simulink model "04_ee_d"  (R2023a)
settings: Solver=VariableStepDiscrete  StartTime=0.0  StopTime=2  RelTol=1e-3  EnableMultiTasking=on
PreLoadFcn:
  | Pnom=100e6;
  | Vnom=35e3;
  | Fnom=50;        %Hz
  | 
  | %DC link
  | Vdc_nom=70e3;       %Volts
  | C_DClink=200e-6; %Farads
  | 
  | %Choke data
  | R_RL=0.10/100;  %pu
  | L_RL=0.10;      %pu
InitFcn:
  | Ts_Power=5e-6;
  | Ts_Control=50e-6;
  | Ts=5e-6;
  | PWM_freq=2600;
undefined symbols (not defined in the file): D11, Delta, DiscIntNeverNeededParam
libraries: spsParallelRLCBranchLib x2, spsThreePhaseVIMeasurementLib x2, spsabctodq0Lib x2, spsSecondOrderFilterLib x2, simulink_extras x2, spsThreePhaseMutualInductanceZ1Z0Lib x1, spsVoltageMeasurementLib x1, spsThreePhaseProgrammableVoltageSourceLib x1, spsThreePhaseTransformerTwoWindingsLib x1, spsDCVoltageSourceLib x1, spsPLL3phLib x1, spsPowerdq0InstantaneousLib x1
settings Model: SimulationMode=accelerator  Creator=Eric  LastModifiedBy=eagle
settings SolverCC: AlgebraicLoopSolver=TrustRegion
settings DataIOCC: SaveFormat=StructureWithTime  SignalLoggingSaveFormat=ModelDataLogs  SaveOutput=off  SignalLogging=off  SaveTime=off  ReturnWorkspaceOutputs=off
settings OptimizationCC: ExpressionDepthLimit=2147483647  InitFltsAndDblsToZero=on  LifeSpan=inf
settings DebuggingCC: SaveWithParameterizedLinksMsg=none  UnderspecifiedInitializationDetection=Classic  MergeDetectMultiDrivingBlocksExec=none  SignalResolutionControl=TryResolveAllWithWarning  SolverPrmCheckMsg=warning  MultiTaskDSMMsg=warning  MultiTaskCondExecSysMsg=none  FcnCallInpInsideContextMsg=warning  AllowSymbolicDim=off  StateNameClashWarn=warning  SFUnexpectedBacktrackingDiag=warning  SFNoUnconditionalDefaultTransitionDiag=warning  SFExecutionAtInitializationDiag=none  ArithmeticOperatorsInVariantConditions=warning
settings HardwareCC: ProdBitPerPointer=32  ProdBitPerSizeT=32  ProdBitPerPtrDiffT=32  ProdLargestAtomicFloat=None  ProdIntDivRoundTo=Undefined  ProdEndianess=Unspecified  ProdWordSize=32  ProdHWDeviceType=32-bit Generic
settings ModelReferenceCC: EnableRefExpFcnMdlSchedulingChecks=on  PropagateSignalLabelsOutOfModel=off
settings SFSimCC: SimUseLocalCustomCode=off  CustomCodeUndefinedFunction=UseInterfaceOnly
settings RTWCC: RTWUseLocalCustomCode=off
settings CodeAppCC: StateflowObjectComments=on
settings GRTTargetCC: TargetFcnLib=ansi_tfl_tmw.mat  TargetLangStandard=C89/C90 (ANSI)  CombineOutputUpdateFcns=off  GRTInterface=on
settings ConfigComp: CovMetricSettings=dw  CovSaveCumulativeToWorkspaceVar=on  CovSaveSingleToWorkspaceVar=on  CovExternalEMLEnable=off  CovSFcnEnable=off
settings SimscapeCC: SimscapeNormalizeSystem=off

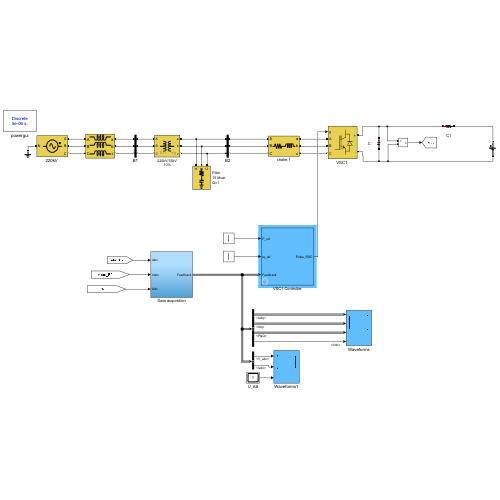
[thumbnail: Simulink's stored preview of the top-level diagram]
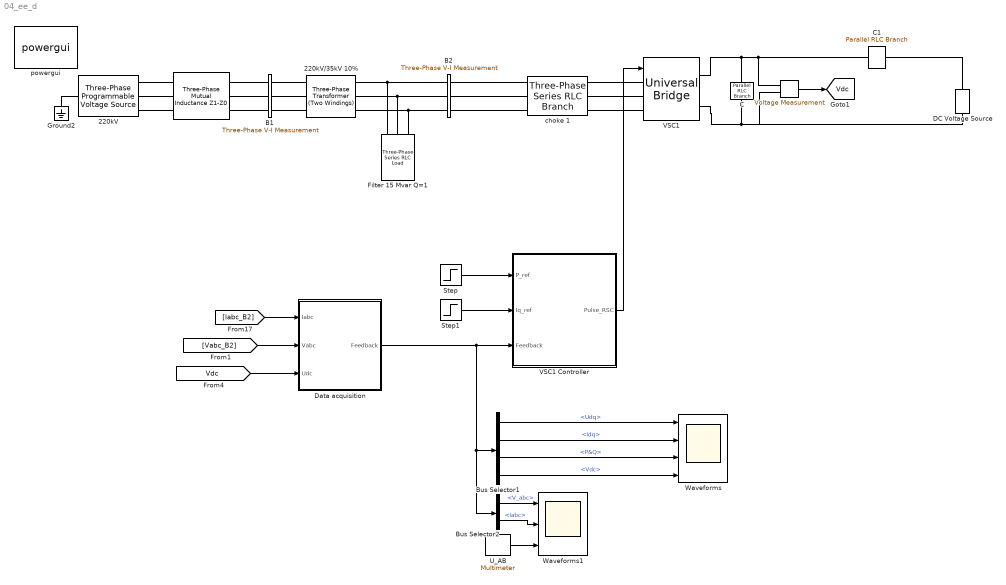
== system 04_ee_d ==
  "  " : spsThreePhaseMutualInductanceZ1Z0Lib/Three-Phase Mutual Inductance Z1-Z0  LConnTagsString=a|b|c  RConnTagsString=A|B|C  PositiveSequence="[ 220e3^2/(10*Pnom)/10  220e3^2/(10*Pnom)/(2*pi*50)]"  ZeroSequence="[220e3^2/(10*Pnom)/10*3  220e3^2/(10*Pnom)/(2*pi*50)*3]"
      settings: AttributesFormatString=\n
      settings: LibrarySourceBlock=|
      | sps_lib/Power Grid Elements/Three-Phase
      | Mutual Inductance
      | Z1-Z0
  "     " : spsVoltageMeasurementLib/Voltage Measurement  PhasorSimulation=off  OutputType=Complex  PSBequivalent=0
  " C" : spsParallelRLCBranchLib/Parallel RLC Branch  LConnTagsString=a  RConnTagsString=__new0  BranchType=C  Resistance=1000000  Inductance=1e-3  SetiL0=off  InitialCurrent=0  Capacitance=C_DClink  Setx0=on  InitialVoltage=Vdc_nom  Measurements=None
  " C1" : spsParallelRLCBranchLib/Parallel RLC Branch  LConnTagsString=a  RConnTagsString=__new0  BranchType=R  Resistance=5  Inductance=1e-3  SetiL0=off  InitialCurrent=0  Capacitance=C_DClink  Setx0=on  InitialVoltage=Vdc_nom  Measurements=None
  "220kV " : spsThreePhaseProgrammableVoltageSourceLib/Three-Phase Programmable Voltage Source  PositiveSequence=[220e3 0 50]  VariationEntity=None  VariationType=Table of time-amplitude pairs  VariationTypeAlt=Step  VariationStep=-0.2  VariationRate=10  VariationMagnitude=0.3  VariationFrequency=2  VariationTiming=[0.05 0.05+5/60]  VariationPhaseA=off  Amplitudes=[1 0.8 1.0]  TimeValues=[0 0.03 0.13]  HarmonicGeneration=off  HarmonicA=[1 0.05 0 2]  HarmonicB=[0 0 0 0]  Timing="[2  20]"  BusType=swing  Pref=0  Qref=0  Qmin=-inf  Qmax=inf
  220kV/35kV 10% : spsThreePhaseTransformerTwoWindingsLib/Three-Phase Transformer (Two Windings)  Winding1Connection=Delta (D11)  Winding2Connection=Yg  CoreType=Three single-phase transformers  SetSaturation=off  Hysteresis=off  DataFile='basic_model'  SetInitialFlux=off  Measurements=None  UNITS=pu  NominalPower=[Pnom*1.5 50 ]  Winding1="[ 220e3  0.05/30   0.05]"  Winding2="[ Vnom 0.05/30  0.05]"  Rm=500  Lm=500  L0=0.5  Saturation="[ 0,0  ;  0.005,1.2  ;  1.0,1.4 ]"  InitialFluxes=[ 0.8 , -0.8 , 0.7 ]  BreakLoop=off  DiscreteSolver=Trapezoidal iterative  DataType=off  TransfoNumber=0
  B1 : spsThreePhaseVIMeasurementLib/Three-Phase V-I Measurement  VoltageMeasurement=phase-to-ground  SetLabelV=on  LabelV=Vabc_B1  Vpu=on  VpuLL=off  CurrentMeasurement=yes  SetLabelI=on  LabelI=Iabc_B1  Ipu=on  Pbase=Pnom  Vbase=220e3  OutputType=Complex  PhasorSimulation=off  PSBequivalent=0
  B2 : spsThreePhaseVIMeasurementLib/Three-Phase V-I Measurement  VoltageMeasurement=phase-to-phase  SetLabelV=on  LabelV=Vabc_B2  Vpu=on  VpuLL=off  CurrentMeasurement=yes  SetLabelI=on  LabelI=Iabc_B2  Ipu=on  Pbase=Pnom  Vbase=Vnom  OutputType=Complex  PhasorSimulation=off  PSBequivalent=0
  Bus Selector1 : BusSelector  OutputSignals=Udq,Idq,P&Q,Vdc
  Bus Selector2 : BusSelector  OutputSignals=V_abc,Iabc
  DC Voltage Source : spsDCVoltageSourceLib/DC Voltage Source  Amplitude=Vdc_nom  Measurements=Voltage
  Data acquisition : Subsystem
  Filter 15 Mvar Q=1 : spsThreePhaseSeriesRLCLoadLib/Three-Phase Series RLC Load  LConnTagsString=A|B|C  Configuration=Y (grounded)  NominalVoltage=Vnom  Vabc=[1e3 1e3 1e3]  Vabcp=[1e3 1e3 1e3]  NominalFrequency=Fnom  UnbalancedPower=off  ActivePower=Pnom*0.15/50  InductivePower=0  CapacitivePower=Pnom*0.15  Pabc=[10e3 9e3 11e3]  QLabc=[100 90 110]  QCabc=[100 90 110]  Pabcp=[10e3 9e3 11e3]  QLabcp=[100 90 110]  QCabcp=[100 90 110]  Measurements=None  LoadType=constant Z
  Ground2 : spsGroundLib/Ground  LConnTagsString=a
  Step : Step  Before=0.5  SampleTime=0
  Step1 : Step  Time=1.5  After=0.2  SampleTime=0
  U_AB : spsMultimeterLib/Multimeter  L=5  sel=1  yselected={}  Gain=1  OutputType=Complex  PlotAtSimulationStop=off  PhasorSimulation=off
  "VSC1 " : spsUniversalBridgeLib/Universal Bridge  Arms=3  SnubberResistance=5000  SnubberCapacitance=1e-6  Device=IGBT / Diodes  Ron=1e-3  Lon=0  ForwardVoltages="[  0  0  ]"  ForwardVoltage=0  GTOparameters=[ 10e-6 , 20e-6 ]  IGBTparameters=[ 0 , 0 ]  Measurements=UAB UBC UCA UDC voltages  Measurements_2=None  converterType=Rectifier
  VSC1 Controller : Subsystem  mask{Kpi_grid_side=[0.5 50 1]}
      mask prompts: Kpi_grid_side "PI controller of Grid-side Current"
      mask init:
      | Kp_grid_side_cur_reg=Kpi_grid_side(1);
      | Ki_grid_side_cur_reg=Kpi_grid_side(2);
      | Limit_U_grid_side=Kpi_grid_side(3);
  Waveforms : Scope  NumInputPorts=4
  Waveforms1 : Scope  NumInputPorts=3
  choke 1 : spsThreePhaseSeriesRLCBranchLib/Three-Phase Series RLC Branch  LConnTagsString=A|B|C  RConnTagsString=A|B|C  BranchType=RL  Resistance=R_RL*Vnom^2/Pnom  Inductance=L_RL*Vnom^2/Pnom/(2*pi*Fnom)  Capacitance=[]  Measurements=None
  powergui : spspowerguiLib/powergui  SimulationMode=Discrete  SampleTime=Ts_Power  frequency=60  Iterations=50  frequencyindice=0  Pbase=100e6  ErrMax=1e-4  UnitsV=kV  UnitsW=MW  buscounter=0  FunctionMessages=off  echomessages=off  EnableUseOfTLC=off  CurrentSourceSwitches=off  DisableSnubberDevices=off  DisableRonSwitches=off  DisableVfSwitches=off  DisplayEquations=off  AutomaticDiscreteSolvers=off  SolverType=Tustin  Interpol=off  ExternalGateDelay=off  methode=off  Ts=0  x0status=blocks  SPID=off  SwTol=0  HookPort=off  NonlinearTolerance=1e-4  nMaxIteration=100  ContinueOnMaxIteration=off  RestoreLinks=warning  ResistiveCurrentMeasurement=off  Frange=[0:2:500]  Ylog=off  Xlog=on  ShowGrid=off  save=off  variable=ZData  structure=AC_Voltage  ZoomFFT=off  StartTime=2  cycles=1  DisplayStyle=5  fundamental=50  FreqAxis=off  MaxFrequency=10000  frequencyindicesteady=1  RmsSteady=1  display=off
  tag scope: Vdc=global
  wires:
  [Iabc_B2] -> Data acquisition/1(Iabc)
  [Vdc] -> Data acquisition/3(Udc)
  Data acquisition/1(Feedback) -> Bus Selector2/1, Bus Selector1/1, VSC1 Controller/3(Feedback)
  [Vabc_B2] -> Data acquisition/2(Vabc)
  Step1/1 -> VSC1 Controller/2(Iq_ref)
  Step/1 -> VSC1 Controller/1(P_ref)
  Bus Selector1/4 -> Waveforms/4  "<Vdc>"
  VSC1 Controller/1(Pulse_RSC) -> "VSC1 "/1
  Bus Selector1/1 -> Waveforms/1  "<Udq>"
  Bus Selector1/2 -> Waveforms/2  "<Idq>"
  Bus Selector1/3 -> Waveforms/3  "<P&Q>"
  "     "/1 -> [Vdc]
  Bus Selector2/1 -> Waveforms1/1  "<V_abc>"
  Bus Selector2/2 -> Waveforms1/2  "<Iabc>"
  U_AB/1 -> Waveforms1/3
  connections:
  Ground2/LConn1 -- "220kV "/LConn1
  B2/RConn1 -- choke 1/LConn1
  B2/RConn2 -- choke 1/LConn2
  B2/RConn3 -- choke 1/LConn3
  choke 1/RConn1 -- "VSC1 "/LConn1
  choke 1/RConn2 -- "VSC1 "/LConn2
  choke 1/RConn3 -- "VSC1 "/LConn3
  "VSC1 "/RConn1 -- " C"/LConn1 -- "     "/LConn1 -- " C1"/LConn1
  220kV/35kV 10%/RConn1 -- Filter 15 Mvar Q=1/LConn1 -- B2/LConn1
  220kV/35kV 10%/RConn2 -- Filter 15 Mvar Q=1/LConn2 -- B2/LConn2
  220kV/35kV 10%/RConn3 -- Filter 15 Mvar Q=1/LConn3 -- B2/LConn3
  "VSC1 "/RConn2 -- "     "/LConn2 -- DC Voltage Source/LConn1 -- " C"/RConn1
  "  "/LConn1 -- "220kV "/RConn1
  "  "/LConn2 -- "220kV "/RConn2
  "  "/LConn3 -- "220kV "/RConn3
  B1/RConn1 -- 220kV/35kV 10%/LConn1
  B1/RConn2 -- 220kV/35kV 10%/LConn2
  B1/RConn3 -- 220kV/35kV 10%/LConn3
  "  "/RConn1 -- B1/LConn1
  "  "/RConn2 -- B1/LConn2
  "  "/RConn3 -- B1/LConn3
  " C1"/RConn1 -- DC Voltage Source/RConn1

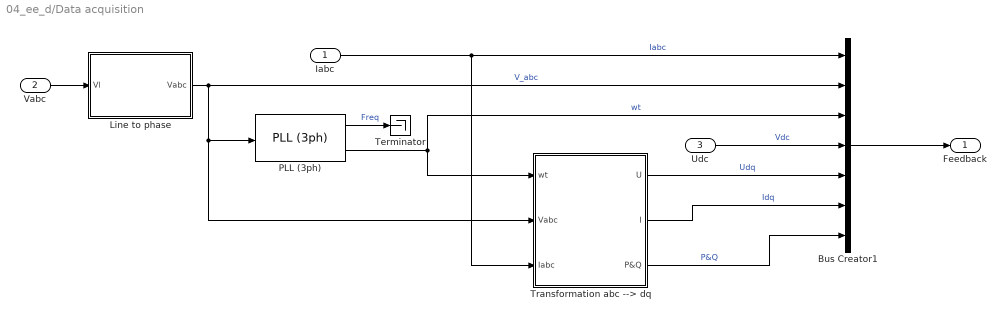
== system 04_ee_d/Data acquisition ==
  Iabc : Inport
  Vabc : Inport  Port=2
  Udc : Inport  Port=3
  Bus Creator1 : BusCreator  Inputs=7
  Line to phase : Subsystem
  PLL (3ph) : spsPLL3phLib/PLL (3ph)  Fmin=45  Par_Init=[0, Fnom]  ParK=[60, 1400]  TcD=0.04  MaxRateChangeFreq=12  FilterCutOffFreq=25  Ts=Ts  AGC=on
  Terminator : Terminator
  Transformation abc --> dq : Subsystem
  Feedback : Outport
  wires:
  Iabc/1 -> Transformation abc --> dq/3(Iabc), Bus Creator1/1  "Iabc"
  Vabc/1 -> Line to phase/1(Vl)
  Bus Creator1/1 -> Feedback/1
  Udc/1 -> Bus Creator1/4  "Vdc"
  Transformation abc --> dq/1(U) -> Bus Creator1/5  "Udq"
  Transformation abc --> dq/2(I) -> Bus Creator1/6  "Idq"
  PLL (3ph)/2 -> Transformation abc --> dq/1(wt), Bus Creator1/3  "wt"
  Line to phase/1(Vabc) -> Transformation abc --> dq/2(Vabc), PLL (3ph)/1, Bus Creator1/2  "V_abc"
  Transformation abc --> dq/3(P&Q) -> Bus Creator1/7  "P&Q"
  PLL (3ph)/1 -> Terminator/1  "Freq"

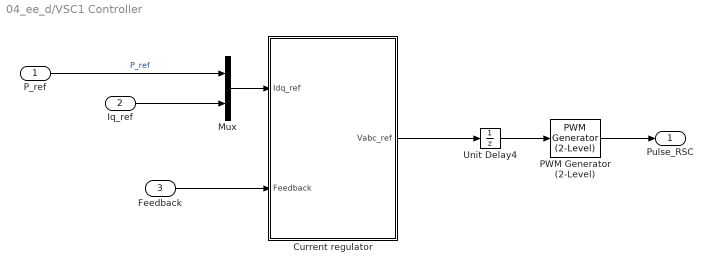
== system 04_ee_d/VSC1 Controller ==
  P_ref : Inport
  Iq_ref : Inport  Port=2
  Feedback : Inport  Port=3
  Current regulator : Subsystem
  Mux : Mux  Inputs=2
  PWM Generator (2-Level) : spsPWMGenerator2LevelLib/PWM Generator (2-Level)  ModulatorType=Three-phase bridge (6 pulses)  ModulatorMode=Unsynchronized  Fc=PWM_freq  Pc=90  nF=27  MinMax="[ -1  1 ]"  SamplingTechnique=Natural  ModulatingSignals=off  m=0.8  Freq=60  Phase=0  Ts=Ts  ShowCarrierOutport=off
  Unit Delay4 : UnitDelay  SampleTime=Ts  HasFrameUpgradeWarning=on
  Pulse_RSC : Outport
  wires:
  Current regulator/1(Vabc_ref) -> Unit Delay4/1
  Unit Delay4/1 -> PWM Generator (2-Level)/1
  Feedback/1 -> Current regulator/2(Feedback)
  PWM Generator (2-Level)/1 -> Pulse_RSC/1
  P_ref/1 -> Mux/1  "P_ref"
  Mux/1 -> Current regulator/1(Idq_ref)
  Iq_ref/1 -> Mux/2

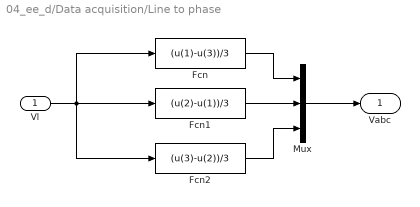
== system 04_ee_d/Data acquisition/Line to phase ==
  Vl : Inport
  Fcn : Fcn  Expr=(u(1)-u(3))/3
  Fcn1 : Fcn  Expr=(u(2)-u(1))/3
  Fcn2 : Fcn  Expr=(u(3)-u(2))/3
  Mux : Mux  Inputs=3
  Vabc : Outport
  wires:
  Fcn/1 -> Mux/1
  Fcn1/1 -> Mux/2
  Mux/1 -> Vabc/1
  Fcn2/1 -> Mux/3
  Vl/1 -> Fcn2/1, Fcn/1, Fcn1/1

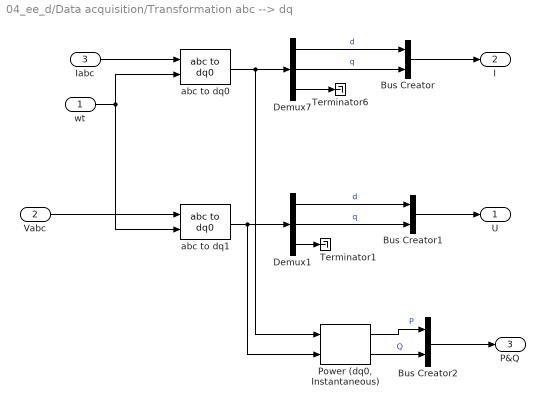
== system 04_ee_d/Data acquisition/Transformation abc --> dq ==
  wt : Inport
  Vabc : Inport  Port=2
  Iabc : Inport  Port=3
  Bus Creator : BusCreator  Inputs=2
  Bus Creator1 : BusCreator  Inputs=2
  Bus Creator2 : BusCreator  Inputs=2
  Demux1 : Demux  Outputs=3
      settings: DisplayOption=none
  Demux7 : Demux  Outputs=3
      settings: DisplayOption=none
  "Power (dq0, Instantaneous)" : spsPowerdq0InstantaneousLib/Power (dq0, Instantaneous)
      settings: LibrarySourceBlock=|
      | sps_lib/Sensors and Measurements/Power
      | (dq0, Instantaneous)
  Terminator1 : Terminator
  Terminator6 : Terminator
  abc to dq0 : spsabctodq0Lib/abc to dq0  Alignment=90 degrees behind phase A axis
  abc to dq1 : spsabctodq0Lib/abc to dq0  Alignment=90 degrees behind phase A axis
  U : Outport
  I : Outport  Port=2
  P&Q : Outport  Port=3
  wires:
  Demux7/2 -> Bus Creator/2  "q"
  Demux7/1 -> Bus Creator/1  "d"
  Bus Creator/1 -> I/1
  Demux7/3 -> Terminator6/1
  abc to dq0/1 -> "Power (dq0, Instantaneous)"/1, Demux7/1
  Iabc/1 -> abc to dq0/1
  Demux1/2 -> Bus Creator1/2  "q"
  Demux1/1 -> Bus Creator1/1  "d"
  Bus Creator1/1 -> U/1
  Demux1/3 -> Terminator1/1
  abc to dq1/1 -> "Power (dq0, Instantaneous)"/2, Demux1/1
  Vabc/1 -> abc to dq1/1
  wt/1 -> abc to dq1/2, abc to dq0/2
  "Power (dq0, Instantaneous)"/1 -> Bus Creator2/1  "P"
  "Power (dq0, Instantaneous)"/2 -> Bus Creator2/2  "Q"
  Bus Creator2/1 -> P&Q/1

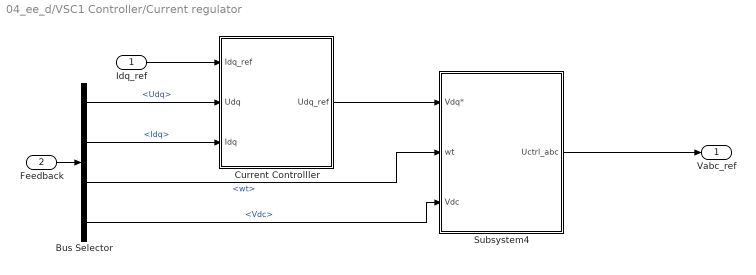
== system 04_ee_d/VSC1 Controller/Current regulator ==
  Idq_ref : Inport
  Feedback : Inport  Port=2
  Bus Selector : BusSelector  OutputSignals=Udq,Idq,wt,Vdc
  Current Controlller : Subsystem
  Subsystem4 : Subsystem
  Vabc_ref : Outport
  wires:
  Bus Selector/4 -> Subsystem4/3(Vdc)  "<Vdc>"
  Bus Selector/3 -> Subsystem4/2(wt)  "<wt>"
  Feedback/1 -> Bus Selector/1
  Subsystem4/1(Uctrl_abc) -> Vabc_ref/1
  Idq_ref/1 -> Current Controlller/1(Idq_ref)
  Bus Selector/1 -> Current Controlller/2(Udq)  "<Udq>"
  Bus Selector/2 -> Current Controlller/3(Idq)  "<Idq>"
  Current Controlller/1(Udq_ref) -> Subsystem4/1(Vdq*)

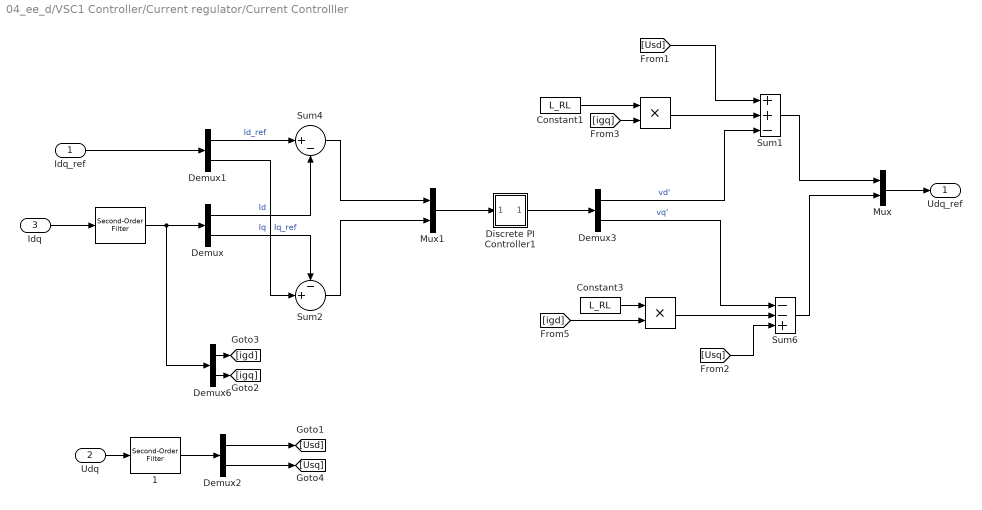
== system 04_ee_d/VSC1 Controller/Current regulator/Current Controlller ==
  Idq_ref : Inport
  Udq : Inport  Port=2
  Idq : Inport  Port=3
  "  " : spsSecondOrderFilterLib/Second-Order Filter  FilterType=Lowpass  Fo=PWM_freq/2  Zeta=0.707  Ts=Ts  Initialize=off  Vac_Init="[0,  0,  60]"  Vdc_Init=0  PlotResponse=off  FreqRange=[0, 500, 1]
      settings: LibrarySourceBlock=|
      | sps_lib/Control/Filters/Second-Order
      | Filter
  "    " : Product  RndMeth=Zero
  "      " : Product  RndMeth=Zero
  "  1" : spsSecondOrderFilterLib/Second-Order Filter  FilterType=Lowpass  Fo=PWM_freq/2  Zeta=0.707  Ts=Ts  Initialize=off  Vac_Init="[0,  0,  60]"  Vdc_Init=0  PlotResponse=off  FreqRange=[0, 500, 1]
      settings: LibrarySourceBlock=|
      | sps_lib/Control/Filters/Second-Order
      | Filter
  Constant1 : Constant  Value=L_RL
  Constant3 : Constant  Value=L_RL
  Demux{,1..3,6} (5 alike) : Demux  Outputs=2
      settings: DisplayOption=none
  Discrete PI Controller1 : Subsystem  AncestorBlock=|  DialogController=POWERSYS.PowerSysDialog  mask(Discrete PI Controller){Kp=Kp_grid_side_cur_reg, Ki=Ki_grid_side_cur_reg, Par_Limits=[1 -1]*Limit_U_grid_side, Init=0, Ts=Ts_Control}
      | powerlib_extras/Discrete 
      | Control Blocks/Discrete
      | PI Controller
      mask prompts: Kp "Proportional gain (Kp):"; Ki "Integral gain (Ki):"; Par_Limits "Output limits: [ Upper   Lower ]"; Init "Output initial value:"; Ts "Sample time:"
      mask help: This block implements a discrete PI controller.
      mask init:
      | UpperLimit=Par_Limits(1);
      | LowerLimit=Par_Limits(2);
      | power_initmask();
      mask Help: This block is part of a subset of blocks in the Extras library that does not have documentation associated with it, other than the block mask description.
      mask Display: disp('PI');
  Mux : Mux  Inputs=2
  Mux1 : Mux  Inputs=2
  Sum1 : Sum  Inputs=++-  InputSameDT=on  SaturateOnIntegerOverflow=on  OutDataTypeStr=Inherit: Same as first input
  Sum2 : Sum  Inputs=-+|  InputSameDT=on  SaturateOnIntegerOverflow=on  OutDataTypeStr=Inherit: Same as first input
  Sum4 : Sum  Inputs=|+-  InputSameDT=on  SaturateOnIntegerOverflow=on  OutDataTypeStr=Inherit: Same as first input
  Sum6 : Sum  Inputs=--+  InputSameDT=on  SaturateOnIntegerOverflow=on  OutDataTypeStr=Inherit: Same as first input
  Udq_ref : Outport
  wires:
  Demux3/2 -> Sum6/1  "vq'"
  Demux1/1 -> Sum4/1  "Id_ref"
  Demux/2 -> Sum2/1  "Iq"
  Demux/1 -> Sum4/2  "Id"
  Sum4/1 -> Mux1/1
  Sum2/1 -> Mux1/2
  Demux3/1 -> Sum1/3  "vd'"
  Mux1/1 -> Discrete PI Controller1/1(Error)
  "      "/1 -> Sum6/2
  Idq_ref/1 -> Demux1/1
  [igd] -> "      "/2
  Constant1/1 -> "    "/1
  [igq] -> "    "/2
  Constant3/1 -> "      "/1
  "    "/1 -> Sum1/2
  Udq/1 -> "  1"/1
  Demux6/1 -> [igd]
  Demux6/2 -> [igq]
  Idq/1 -> "  "/1
  Sum1/1 -> Mux/1
  Sum6/1 -> Mux/2
  Demux1/2 -> Sum2/2  "Iq_ref"
  "  "/1 -> Demux6/1, Demux/1
  Discrete PI Controller1/1(Out) -> Demux3/1
  Mux/1 -> Udq_ref/1
  "  1"/1 -> Demux2/1
  Demux2/1 -> [Usd]
  Demux2/2 -> [Usq]
  [Usd] -> Sum1/1
  [Usq] -> Sum6/3

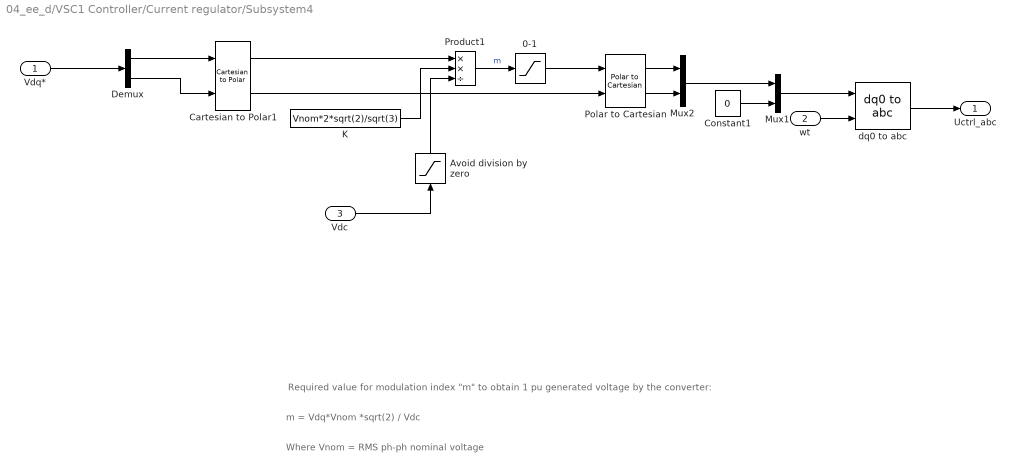
== system 04_ee_d/VSC1 Controller/Current regulator/Subsystem4 ==
  note: Where Vnom = RMS ph-ph nominal voltage
  note: m = Vdq*Vnom *sqrt(2) / Vdc
  note: Required value for modulation index "m" to obtain 1 pu generated voltage by the converter:
  Vdq* : Inport
  wt : Inport  Port=2
  Vdc : Inport  Port=3
  0-1 : Saturate  UpperLimit=1  LowerLimit=0
  Avoid division by zero : Saturate  UpperLimit=Vdc_nom*2  LowerLimit=10
  Cartesian to Polar1 : simulink_extras/Transformations/Cartesian to Polar
  Constant1 : Constant  Value=0
  Demux : Demux  Outputs=2
  K : Constant  Value=Vnom*2*sqrt(2)/sqrt(3)
  Mux1 : Mux  Inputs=[2 1]
  Mux2 : Mux  Inputs=2
  Polar to Cartesian : simulink_extras/Transformations/Polar to Cartesian
  Product1 : Product  Inputs=**/  InputSameDT=on  SaturateOnIntegerOverflow=on  OutDataTypeStr=Inherit: Same as first input
  dq0 to abc : spsdq0toabcLib/dq0 to abc  Alignment=90 degrees behind phase A axis
  Uctrl_abc : Outport
  wires:
  Polar to Cartesian/2 -> Mux2/2
  Polar to Cartesian/1 -> Mux2/1
  Vdq*/1 -> Demux/1
  Cartesian to Polar1/2 -> Polar to Cartesian/2
  Cartesian to Polar1/1 -> Product1/1
  Avoid division by zero/1 -> Product1/3
  K/1 -> Product1/2
  Product1/1 -> 0-1/1  "m"
  0-1/1 -> Polar to Cartesian/1
  Demux/2 -> Cartesian to Polar1/2
  Demux/1 -> Cartesian to Polar1/1
  dq0 to abc/1 -> Uctrl_abc/1
  Mux1/1 -> dq0 to abc/1
  Constant1/1 -> Mux1/2
  Mux2/1 -> Mux1/1
  wt/1 -> dq0 to abc/2
  Vdc/1 -> Avoid division by zero/1

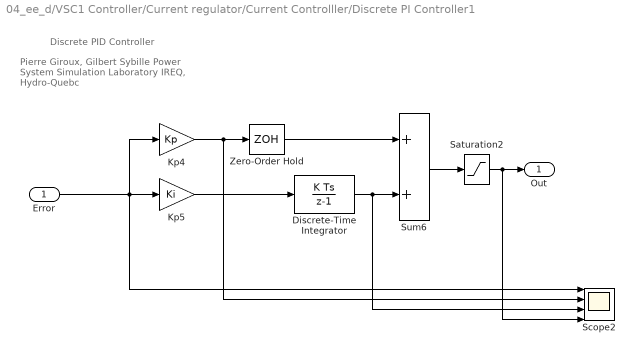
== system 04_ee_d/VSC1 Controller/Current regulator/Current Controlller/Discrete PI Controller1 ==
  note: Discrete PID Controller
  note: Pierre Giroux, Gilbert Sybille
      | Power System Simulation Laboratory
      | IREQ, Hydro-Quebc
  Error : Inport  SampleTime=Ts
  Discrete-Time Integrator : DiscreteIntegrator  InitialCondition=Init  SampleTime=Ts  LimitOutput=on  UpperSaturationLimit=UpperLimit  LowerSaturationLimit=LowerLimit  ICPrevOutput=DiscIntNeverNeededParam  ICPrevScaledInput=DiscIntNeverNeededParam
  Kp4 : Gain  Gain=Kp  SaturateOnIntegerOverflow=on  SampleTime=Ts  OutDataTypeStr=Inherit: Same as input  ParamDataTypeStr=Inherit: Same as input
  Kp5 : Gain  Gain=Ki  SaturateOnIntegerOverflow=on  SampleTime=Ts  OutDataTypeStr=Inherit: Same as input  ParamDataTypeStr=Inherit: Same as input
  Saturation2 : Saturate  UpperLimit=UpperLimit  LowerLimit=LowerLimit  SampleTime=Ts
  Scope2 : Scope  NumInputPorts=4
  Sum6 : Sum  InputSameDT=on  SaturateOnIntegerOverflow=on  SampleTime=Ts  OutDataTypeStr=Inherit: Same as first input
  Zero-Order Hold : ZeroOrderHold  SampleTime=Ts
  Out : Outport  SampleTime=Ts  InitialOutput=0
  wires:
  Zero-Order Hold/1 -> Sum6/1
  Saturation2/1 -> Scope2/4, Out/1
  Discrete-Time Integrator/1 -> Scope2/3, Sum6/2
  Kp4/1 -> Scope2/2, Zero-Order Hold/1
  Kp5/1 -> Discrete-Time Integrator/1
  Sum6/1 -> Saturation2/1
  Error/1 -> Scope2/1, Kp5/1, Kp4/1
